simulink model "simulink"  (R2020b)
settings: Solver=VariableStepAuto  StartTime=0.0  StopTime=10.0  RelTol=1e-3
settings Model: Creator=amirh  LastModifiedBy=amirh

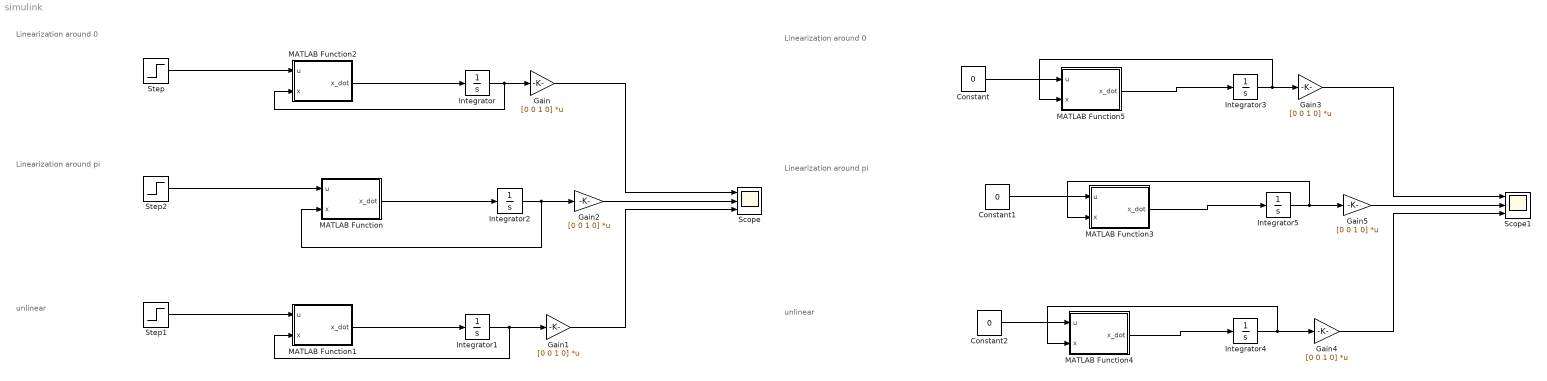
== system simulink ==
  note: Linearization around 0
  note: Linearization around pi
  note: unlinear
  note: unlinear
  note: Linearization around pi
  note: Linearization around 0
  Constant : Constant  Value=0
  Constant1 : Constant  Value=0
  Constant2 : Constant  Value=0
  Gain{,1..5} (6 alike) : Gain  Gain=[0 0 1 0]  Multiplication=Matrix(K*u)
  Integrator : Integrator  InitialCondition=zeros(4,1)
  Integrator1 : Integrator  InitialCondition=zeros(4,1)
  Integrator2 : Integrator  InitialCondition=[pi;0;pi;0]
  Integrator3 : Integrator  InitialCondition=[1 0 1 0]
  Integrator4 : Integrator  InitialCondition=[1 0 1 0]
  Integrator5 : Integrator  InitialCondition=[1 0 1 0]
  MATLAB Function : MATLAB Function  TreatAsAtomicUnit=on
  MATLAB Function1 : MATLAB Function  TreatAsAtomicUnit=on
  MATLAB Function2 : MATLAB Function  TreatAsAtomicUnit=on
  MATLAB Function3 : MATLAB Function  TreatAsAtomicUnit=on
  MATLAB Function4 : MATLAB Function  TreatAsAtomicUnit=on
  MATLAB Function5 : MATLAB Function  TreatAsAtomicUnit=on
  Scope : Scope  NumInputPorts=3
  Scope1 : Scope  NumInputPorts=3
  Step : Step  SampleTime=0
  Step1 : Step  After=0.02  SampleTime=0
  Step2 : Step  SampleTime=0
  wires:
  Step2/1 -> MATLAB Function/1(u)
  Step1/1 -> MATLAB Function1/1(u)
  Step/1 -> MATLAB Function2/1(u)
  MATLAB Function/1(x_dot) -> Integrator2/1
  Integrator2/1 -> MATLAB Function/2(x), Gain2/1
  MATLAB Function1/1(x_dot) -> Integrator1/1
  MATLAB Function2/1(x_dot) -> Integrator/1
  Integrator1/1 -> Gain1/1, MATLAB Function1/2(x)
  Integrator/1 -> Gain/1, MATLAB Function2/2(x)
  Gain/1 -> Scope/1
  Gain1/1 -> Scope/3
  Gain2/1 -> Scope/2
  Gain5/1 -> Scope1/2
  MATLAB Function4/1(x_dot) -> Integrator4/1
  MATLAB Function3/1(x_dot) -> Integrator5/1
  Integrator3/1 -> Gain3/1, MATLAB Function5/2(x)
  Gain3/1 -> Scope1/1
  Gain4/1 -> Scope1/3
  MATLAB Function5/1(x_dot) -> Integrator3/1
  Integrator4/1 -> Gain4/1, MATLAB Function4/2(x)
  Integrator5/1 -> MATLAB Function3/2(x), Gain5/1
  Constant/1 -> MATLAB Function5/1(u)
  Constant2/1 -> MATLAB Function4/1(u)
  Constant1/1 -> MATLAB Function3/1(u)

== matlab function simulink/MATLAB Function ==
  data: u input; x_dot output; x input
function x_dot = fcn(u,x)

A=[-0.0297    1.1746   -0.0000   -0.0000;
   -1.1746   -0.0297    0.0000    0.0000;
   -0.0000   -0.0000   -0.0295    1.3250;
    0.0000    0.0000   -1.3250   -0.0295];
B=[ 27.0158;
   -0.6643;
    0.4482;
   -0.0324];

x_dot = A*x +B*u

== matlab function simulink/MATLAB Function2 ==
  data: u input; x_dot output; x input
function x_dot = fcn(u,x)

A=[-0.0297    1.1746   -0.0000   -0.0000;
   -1.1746   -0.0297    0.0000    0.0000;
   -0.0000   -0.0000   -0.0295    1.3250;
    0.0000    0.0000   -1.3250   -0.0295];
B=[ 27.0158;
   -0.6643;
    0.4482;
   -0.0324];

x_dot = A*x +B*u

== matlab function simulink/MATLAB Function3 ==
  data: u input; x_dot output; x input
function x_dot = fcn(u,x)

A=[-0.0297    1.1746   -0.0000   -0.0000;
   -1.1746   -0.0297    0.0000    0.0000;
   -0.0000   -0.0000   -0.0295    1.3250;
    0.0000    0.0000   -1.3250   -0.0295];
B=[ 27.0158;
   -0.6643;
    0.4482;
   -0.0324];

x_dot = A*x +B*u

== matlab function simulink/MATLAB Function4 ==
  data: u input; x_dot output; x input
function x_dot = fcn(u,x)
theta1=x(1);
theta1_d=x(2);
theta2=x(3);
theta2_d=x(4);

theta1_dd=(2*cos(theta1 - theta2)*sin(theta1 - theta2)*theta1_d^2 + 1890*theta1_d + 252*sin(theta1 - theta2)*theta2_d^2 - 15*cos(theta1 - theta2)*theta2_d + 31500*theta1 + 24696*sin(theta1) - 98*cos(theta1 - theta2)*sin(theta2) - 250*theta2*cos(theta1 - theta2))/(2*(cos(theta1 - theta2)^2 - 16002)) - (1601*u)/100;
theta2_dd=(971*u)/25 - (254*sin(theta1 - theta2)*theta1_d^2 + 15*cos(theta1 - theta2)*theta1_d + 2*cos(theta1 - theta2)*sin(theta1 - theta2)*theta2_d^2 - 1905*theta2_d - 31750*theta2 - 12446*sin(theta2) + 196*cos(theta1 - theta2)*sin(theta1) + 250*theta1*cos(theta1 - theta2))/(2*(cos(theta1 - theta2)^2 - 16002));
 
x_dot=zeros(4,1);
x_dot(1)=theta1_d;
x_dot(2) =theta1_dd;
x_dot(3)=theta2_d;
x_dot(4)=theta2_dd;

== matlab function simulink/MATLAB Function5 ==
  data: u input; x_dot output; x input
function x_dot = fcn(u,x)

A=[-0.0297    1.1746   -0.0000   -0.0000;
   -1.1746   -0.0297    0.0000    0.0000;
   -0.0000   -0.0000   -0.0295    1.3250;
    0.0000    0.0000   -1.3250   -0.0295];
B=[ 27.0158;
   -0.6643;
    0.4482;
   -0.0324];

x_dot = A*x +B*u

== matlab function simulink/MATLAB Function1 ==
  data: u input; x_dot output; x input
function x_dot = fcn(u,x)
theta1=x(1);
theta1_d=x(2);
theta2=x(3);
theta2_d=x(4);

theta1_dd=(2*cos(theta1 - theta2)*sin(theta1 - theta2)*theta1_d^2 + 1890*theta1_d + 252*sin(theta1 - theta2)*theta2_d^2 - 15*cos(theta1 - theta2)*theta2_d + 31500*theta1 + 24696*sin(theta1) - 98*cos(theta1 - theta2)*sin(theta2) - 250*theta2*cos(theta1 - theta2))/(2*(cos(theta1 - theta2)^2 - 16002)) - (1601*u)/100;
theta2_dd=(971*u)/25 - (254*sin(theta1 - theta2)*theta1_d^2 + 15*cos(theta1 - theta2)*theta1_d + 2*cos(theta1 - theta2)*sin(theta1 - theta2)*theta2_d^2 - 1905*theta2_d - 31750*theta2 - 12446*sin(theta2) + 196*cos(theta1 - theta2)*sin(theta1) + 250*theta1*cos(theta1 - theta2))/(2*(cos(theta1 - theta2)^2 - 16002));
 
x_dot=zeros(4,1);
x_dot(1)=theta1_d;
x_dot(2) =theta1_dd;
x_dot(3)=theta2_d;
x_dot(4)=theta2_dd;
